simulink model "dsplpc"  (Simulink 8.3)
settings: Solver=FixedStepDiscrete  SolverMode=SingleTasking  StartTime=0.0  StopTime=5  RelTol=1e-3
PostLoadFcn:
  | open_system('dsplpc/LPC Analysis/LPC Spectrum')
model workspace: external: MAT-File mtlb.mat (data not in the file)
undefined symbols (not defined in the file or in its folder): dfilt, Mag
libraries: dsparch4 x4, dspsnks4 x2, dspsigops x2, dspvision x1, dspmisc x1, dspstat3 x1, dspxfrm3 x1, dspsolvers x1
settings Model: RequirementInfo=9  Creator=The MathWorks Inc.  ExtModeTrigMode=oneshot  ExtModeArmWhenConnect=off
settings DataIOCC: LimitDataPoints=off  SaveOutput=off  SaveTime=off  SignalLoggingName=sigsOut
settings OptimizationCC: BlockReduction=off  BooleanDataType=off  ExpressionDepthLimit=2147483647  InitFltsAndDblsToZero=on
settings DebuggingCC: SignalResolutionControl=TryResolveAllWithWarning  SolverPrmCheckMsg=none  MultiTaskDSMMsg=warning  MultiTaskCondExecSysMsg=none  SingleTaskRateTransMsg=error  IntegerOverflowMsg=none  FcnCallInpInsideContextMsg=UseLocalSettings
settings HardwareCC: ProdHWDeviceType=Specified
settings RTWCC: IncludeERTFirstTime=on
settings GRTTargetCC: TargetFcnLib=ansi_tfl_tmw_new.mat

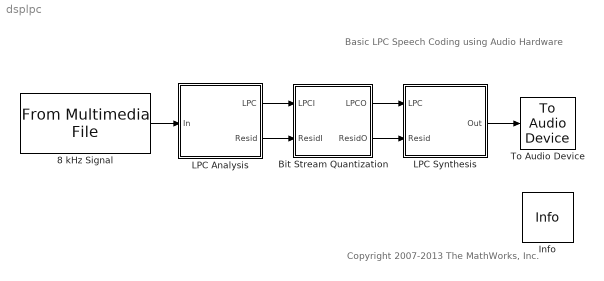
== system dsplpc ==
  note: Basic LPC Speech Coding using Audio Hardware
  note: Copyright 2007-2013 The MathWorks, Inc.
  8 kHz Signal : dspvision/From Multimedia File  inputFilename=speech_dft_8kHz.wav  loop=on  numPlays=1  outputStreams=Audio only  videoDataType=single  audioDataType=double  inheritSampleTime=on  userDefinedSampleTime=1/30  noAudioOutput=off  isIntensityVideo=off  fourcc=RGB  colorVideoFormat=Separate color signals  outputEOF=off  dataOrg=Column-major  audioFrameSize=80  computeAudioFrameSize=off  outSamplingMode=Frame based
  Bit Stream Quantization : Subsystem
  Info : dspmisc/Info  SystemSampleTime=-1
  LPC Analysis : Subsystem
  LPC Synthesis : Subsystem
  To Audio Device : dspsnks4/To Audio Device  deviceName=Default  inheritSampleRate=on  sampleRate=44100  deviceDatatype=Determine from input data type  autoBufferSize=on  bufferSize=4096  queueDuration=0.2  defaultOutputChannelMapping=on  outputChannelMapping=1
  wires:
  LPC Analysis/1(LPC) -> Bit Stream Quantization/1(LPCI)
  LPC Analysis/2(Resid) -> Bit Stream Quantization/2(ResidI)
  8 kHz Signal/1 -> LPC Analysis/1(In)
  Bit Stream Quantization/2(ResidO) -> LPC Synthesis/2(Resid)
  Bit Stream Quantization/1(LPCO) -> LPC Synthesis/1(LPC)
  LPC Synthesis/1(Out) -> To Audio Device/1

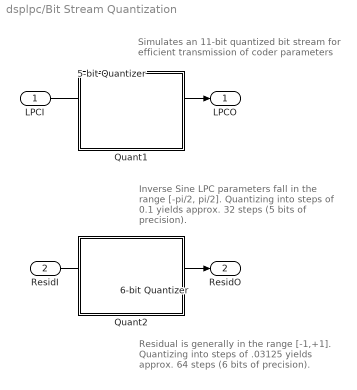
== system dsplpc/Bit Stream Quantization ==
  note: Inverse Sine LPC parameters fall in
      | the range [-pi/2, pi/2].  Quantizing
      | into steps of 0.1 yields approx. 32 steps
      | (5 bits of precision).
  note: Residual is generally in the range [-1,+1].
      | Quantizing into steps of .03125 yields
      | approx. 64 steps (6 bits of precision).
  note: Simulates an 11-bit quantized bit stream
      | for efficient transmission of coder parameters
  LPCI : Inport
  ResidI : Inport  Port=2
  5-bit Quantizer : Quantizer  QuantizationInterval=0.1  LinearizeAsGain=off
  6-bit Quantizer : Quantizer  QuantizationInterval=0.03125  LinearizeAsGain=off
  Quant1 : Subsystem
      mask Display: disp('')
  Quant2 : Subsystem
      mask Display: disp('')
  LPCO : Outport
  ResidO : Outport  Port=2
  wires:
  6-bit Quantizer/1 -> ResidO/1
  ResidI/1 -> 6-bit Quantizer/1
  5-bit Quantizer/1 -> LPCO/1
  LPCI/1 -> 5-bit Quantizer/1

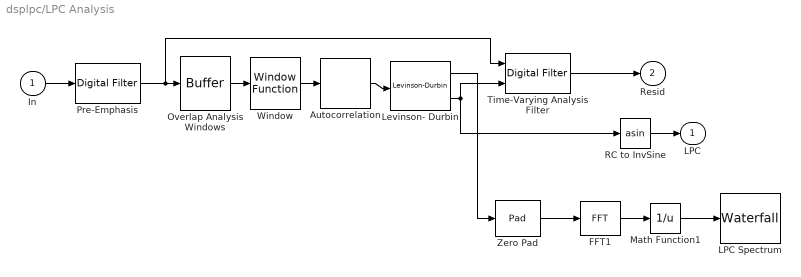
== system dsplpc/LPC Analysis ==
  In : Inport
  Autocorrelation : dspstat3/Autocorrelation  AllPositiveLags=off  maxlag=10  bias=Biased  domain=Time  outputMin=[]  outputMax=[]  accumDataTypeStr=Inherit: Same as product output  accumLastDataTypeStr=Inherit: Same as product output  roundingMode=Floor  overflowMode=off
  FFT1 : dspxfrm3/FFT  CompMethod=Table lookup  TableOpt=NEW  TableOptActive=Speed  BitRevOrder=off  InheritFFTLength=on  FFTLength=64  WrapInput=on  RowConvenienceOn=on  FFTImplementation=Auto  SkipNorm=off  firstCoeffDataTypeStr=Inherit: Same word length as input  firstCoeffLastDataTypeStr=Inherit: Same word length as input  outputMin=[]  outputMax=[]  accumDataTypeStr=Inherit: Same as product output  accumLastDataTypeStr=Inherit: Same as product output  roundingMode=Floor  overflowMode=off
  LPC Spectrum : dspsnks4/Waterfall  TraceProperties=off  NumTraces=10  CMapStr=autumn  TNewest=0.7  TOldest=0.1  HistoryLength=50  HistoryFull=Overwrite  UpdateInterval=1  ExportMode=All visible  MLExportName=ExportData  AutoExport=off  DisplayProperties=off  MouseMode=Orbit  AxisGrid=on  Snapshot=off  Suspend=off  SyncSnapshots=off  OpenScopeAtSimStart=on  FigPos=[35 341 410 358]  CameraView=[89945.9047576273 49093.2447020758 -7462.52930692949 -16.6995606364064 71 5.5 2.5389885178677 -5.30668596526891 0.808418434368868 0.0592442608385446 5.583225828012 14.2 1]  InportDimsHint=[129 1]  AxisProperties=off  AxisColor=[1 1 1]*.9  XLabel=Frequency  YLabel=Mag^2  ZLabel=History  TriggerProperties=off  TrigStartMode=Immediately  TrigStartT=10  TrigStartN=1000  TrigStartFcn=trigPower  TrigStopMode=Never  TrigStopT=0.1  TrigStopN=10  TrigStopFcn=trigend  TrigRearmMode=User-defined  TrigRearmT=0  TrigRearmN=100  TrigRearmFcn=trigrearm  XformProperties=off  XformMode=FFT->Mag dB Fs/2  XformFcn=fliplr  XformExpr=20*log10(abs(u(129:2:end)))
      settings: YMin=-44.6156897764664  YMax=28
  Levinson- Durbin : dspsolvers/Levinson-Durbin  coeffOutFcn=OBSOLETE  coeffOutFcnActive=A and K  outP=off  zeroInpHandling=on  firstCoeffMode=Binary point scaling  firstCoeffWordLength=16  firstCoeffFracLength=15  firstCoeffDataTypeStr=fixdt(1,16,15)  firstCoeffLastDataTypeStr=fixdt(1,16,15)  firstCoeffMin=[]  firstCoeffMax=[]  secondCoeffMode=Binary point scaling  secondCoeffWordLength=16  secondCoeffFracLength=15  secondCoeffDataTypeStr=fixdt(1,16,15)  secondCoeffLastDataTypeStr=fixdt(1,16,15)  secondCoeffMin=[]  secondCoeffMax=[]  outputMin=[]  outputMax=[]  roundingMode=Floor  overflowMode=off
      settings: allowOverrides=off
  Math Function1 : Math  Operator=reciprocal  SaturateOnIntegerOverflow=on
  Overlap Analysis Windows : Buffer  N=160  V=80  TreatMby1Signals=One channel
  Pre-Emphasis : dsparch4/Digital Filter  TypePopup=FIR (all zeros)  IIRFiltStruct=Direct form II transposed  AllPoleFiltStruct=Direct form  FIRFiltStruct=Direct form  CoeffSource=Specify via dialog  NumCoeffs=[1 -.95]  DenCoeffs=[1 0.1]  BiQuadCoeffs=[1 0.3 0.4 1 0.1 0.2]  LatticeCoeffs=[0.2 0.4]  denIgnore=on  FiltPerSampPopup=One filter per frame  IC=0  ICnum=0  ICden=0  roundingMode=Floor  overflowMode=off  ScaleValues=1  scaleValueFracLength=14  stageInFracLength=15  stageOutFracLength=15  FilterSource=Specify via dialog  dfiltObjectName=dfilt.dffir([1 2 1])  InputProcessing=Columns as channels (frame based)
  RC to InvSine : Trigonometry  Operator=asin
  Time-Varying Analysis Filter : dsparch4/Digital Filter  TypePopup=FIR (all zeros)  IIRFiltStruct=Direct form II transposed  AllPoleFiltStruct=Direct form  FIRFiltStruct=Lattice MA  CoeffSource=Input port(s)  NumCoeffs=[1 -.95] / 3.0  DenCoeffs=[1 0.1]  BiQuadCoeffs=[1 0.3 0.4 1 0.1 0.2]  LatticeCoeffs=[0.2 0.4]  denIgnore=on  FiltPerSampPopup=One filter per frame  IC=0  ICnum=0  ICden=0  roundingMode=Floor  overflowMode=off  ScaleValues=1  scaleValueFracLength=14  stageInFracLength=15  stageOutFracLength=15  FilterSource=Input port(s)  dfiltObjectName=dfilt.dffir([1 2 1])  InputProcessing=Columns as channels (frame based)
  Window : dspsigops/Window Function  winmode=Apply window to input  wintype=Hamming  sampmode=Continuous  samptime=1  N=64  Rs=50  beta=10  winsamp=Symmetric  UserWindow=hamming  OptParams=off  UserParams={1.0}  RowConvenienceOn=on  dataType=double  isSigned=on  wordLen=16  udDataType=sfix(16)  fracBitsMode=Best precision  numFracBits=15  roundingMode=Floor  overflowMode=off  numSidelobes=4  sidelobeLevel=-30
  Zero Pad : dspsigops/Pad  padAlong=Columns  dimsToPad=1  valSrc=Specify via dialog  padVal=0  spec=Output size  padNumOutRowsSpecMethod=User-specified  numOutRows=256  padNumOutColsSpecMethod=User-specified  numOutCols=1  isVarDimsMode=off  padBeginning=0  padEnd=0  outSizeMode=User-specified  outSize=1  padSigAt=End  trunc_flag=None  roundingMode=Floor  overflowMode=off  truncOrWrapMode=Truncate  wrap_flag=None
  LPC : Outport
  Resid : Outport  Port=2
  wires:
  Pre-Emphasis/1 -> Overlap Analysis Windows/1, Time-Varying Analysis Filter/1
  Overlap Analysis Windows/1 -> Window/1
  Autocorrelation/1 -> Levinson- Durbin/1
  Window/1 -> Autocorrelation/1
  Levinson- Durbin/2 -> Time-Varying Analysis Filter/2, RC to InvSine/1
  RC to InvSine/1 -> LPC/1
  In/1 -> Pre-Emphasis/1
  Time-Varying Analysis Filter/1 -> Resid/1
  Zero Pad/1 -> FFT1/1
  FFT1/1 -> Math Function1/1
  Math Function1/1 -> LPC Spectrum/1
  Levinson- Durbin/1 -> Zero Pad/1

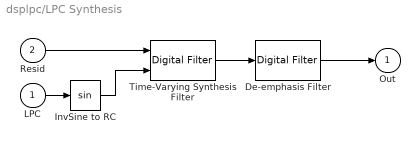
== system dsplpc/LPC Synthesis ==
  LPC : Inport
  Resid : Inport  Port=2
  De-emphasis Filter : dsparch4/Digital Filter  TypePopup=IIR (all poles)  IIRFiltStruct=Direct form II transposed  AllPoleFiltStruct=Direct form  FIRFiltStruct=Direct form  CoeffSource=Specify via dialog  NumCoeffs=[1 -.95] / 3.0  DenCoeffs=[1 -.95]  BiQuadCoeffs=[1 0.3 0.4 1 0.1 0.2]  LatticeCoeffs=[0.2 0.4]  denIgnore=on  FiltPerSampPopup=One filter per frame  IC=0  ICnum=0  ICden=0  roundingMode=Floor  overflowMode=off  ScaleValues=1  scaleValueFracLength=14  stageInFracLength=15  stageOutFracLength=15  FilterSource=Specify via dialog  dfiltObjectName=dfilt.dffir([1 2 1])  InputProcessing=Columns as channels (frame based)
  InvSine to RC : Trigonometry
  Time-Varying Synthesis Filter : dsparch4/Digital Filter  TypePopup=IIR (all poles)  IIRFiltStruct=Direct form II transposed  AllPoleFiltStruct=Lattice AR  FIRFiltStruct=Direct form  CoeffSource=Input port(s)  NumCoeffs=[1 -.95] / 3.0  DenCoeffs=[1 0.1]  BiQuadCoeffs=[1 0.3 0.4 1 0.1 0.2]  LatticeCoeffs=[0.2 0.4]  denIgnore=on  FiltPerSampPopup=One filter per frame  IC=0  ICnum=0  ICden=0  roundingMode=Floor  overflowMode=off  ScaleValues=1  scaleValueFracLength=14  stageInFracLength=15  stageOutFracLength=15  FilterSource=Input port(s)  dfiltObjectName=dfilt.dffir([1 2 1])  InputProcessing=Columns as channels (frame based)
  Out : Outport
  wires:
  Time-Varying Synthesis Filter/1 -> De-emphasis Filter/1
  Resid/1 -> Time-Varying Synthesis Filter/1
  LPC/1 -> InvSine to RC/1
  InvSine to RC/1 -> Time-Varying Synthesis Filter/2
  De-emphasis Filter/1 -> Out/1

== system dsplpc/Bit Stream Quantization/Quant1 ==

== system dsplpc/Bit Stream Quantization/Quant2 ==
